simulink model "prelim_plant"  (R2017b)
settings: Solver=VariableStepAuto  StartTime=0.0  StopTime=100  RelTol=1e-3  EnableMultiTasking=on
undefined symbols (not defined in the file or in its folder): A_nom, B_nom, C, D
libraries: cstblocks x6
settings Model: Creator=yyakupog  LastModifiedBy=USER
settings OptimizationCC: LifeSpan=inf
settings DebuggingCC: SFUnexpectedBacktrackingDiag=warning  SFNoUnconditionalDefaultTransitionDiag=warning  SFExecutionAtInitializationDiag=none
settings CodeAppCC: StateflowObjectComments=on
settings GRTTargetCC: TargetLangStandard=C89/C90 (ANSI)  GeneratePreprocessorConditionals=Disable all
settings ConfigComp: CovMetricSettings=dw  CovHtmlReporting=on  CovSaveCumulativeToWorkspaceVar=on  CovSaveSingleToWorkspaceVar=on  CovExternalEMLEnable=off

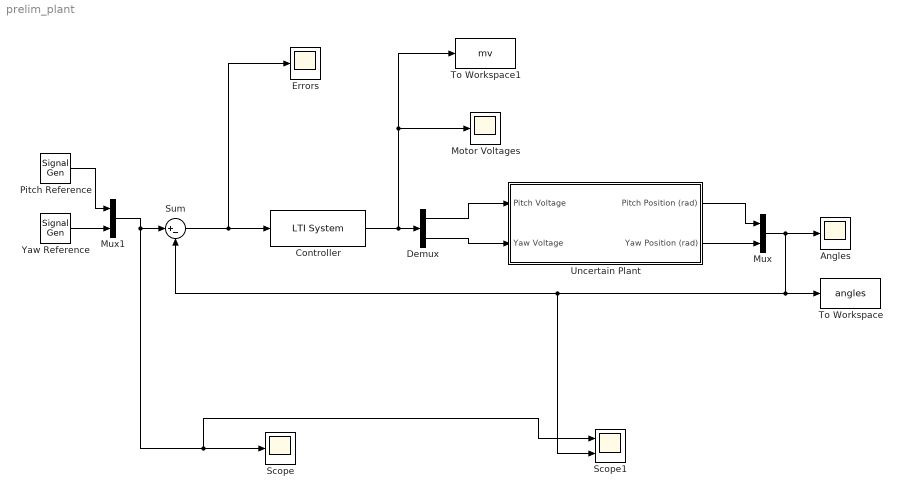
== system prelim_plant ==
  Angles : Scope
  Controller : cstblocks/LTI System  sys=K  IC=[]
  Demux : Demux  Outputs=2
  Errors : Scope
  Motor Voltages : Scope
  Mux : Mux  Inputs=2
  Mux1 : Mux  Inputs=2
  "Pitch Reference " : SignalGenerator  WaveForm=square  Amplitude=pi/6  Frequency=0.4  Units=rad/sec
  Scope : Scope
  Scope1 : Scope  NumInputPorts=2
  Sum : Sum  Inputs=|+-
  To Workspace : ToWorkspace  VariableName=angles  SaveFormat=Timeseries  SampleTime=-1
  To Workspace1 : ToWorkspace  VariableName=mv  SaveFormat=Timeseries  SampleTime=-1
  Uncertain Plant : Subsystem
  Yaw Reference : SignalGenerator  WaveForm=square  Amplitude=pi/4  Frequency=0.5  Units=rad/sec
  wires:
  Controller/1 -> To Workspace1/1, Motor Voltages/1, Demux/1
  Demux/1 -> Uncertain Plant/1(Pitch Voltage)
  Demux/2 -> Uncertain Plant/2(Yaw Voltage)
  Sum/1 -> Errors/1, Controller/1
  Uncertain Plant/1(Pitch Position (rad)) -> Mux/1
  Uncertain Plant/2(Yaw Position (rad)) -> Mux/2
  "Pitch Reference "/1 -> Mux1/1
  Yaw Reference/1 -> Mux1/2
  Mux1/1 -> Scope1/1, Scope/1, Sum/1
  Mux/1 -> To Workspace/1, Scope1/2, Sum/2, Angles/1

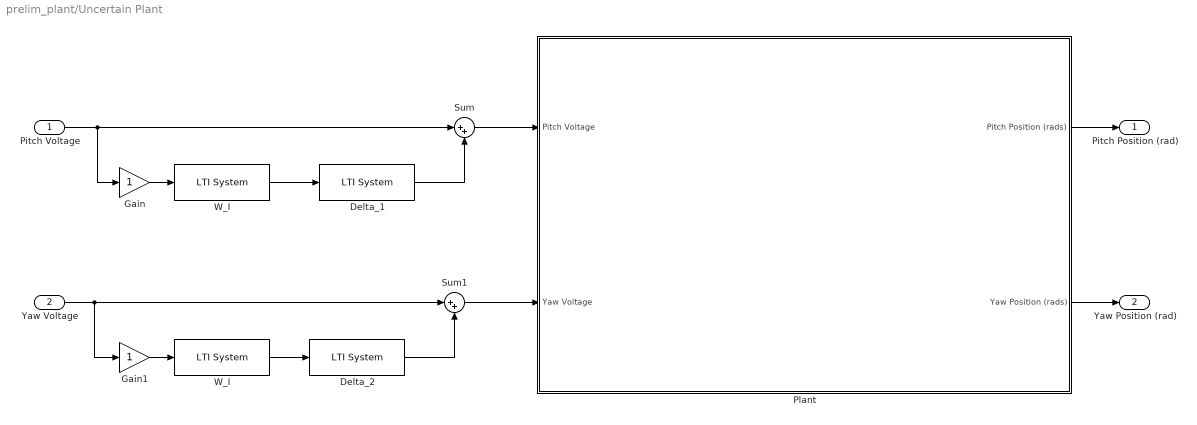
== system prelim_plant/Uncertain Plant ==
  Pitch Voltage : Inport
  Yaw Voltage : Inport  Port=2
  Delta_1 : cstblocks/LTI System  sys=Delta_1  IC=[]
  Delta_2 : cstblocks/LTI System  sys=Delta_2  IC=[]
  Gain : Gain
  Gain1 : Gain
  Plant : Subsystem
  Sum : Sum  Inputs=|++
  Sum1 : Sum  Inputs=|++
  W_I : cstblocks/LTI System  sys=W_I_Pitch  IC=[]
  "W_I " : cstblocks/LTI System  sys=W_I_Yaw  IC=[]
  Pitch Position (rad) : Outport
  Yaw Position (rad) : Outport  Port=2
  wires:
  W_I/1 -> Delta_1/1
  Pitch Voltage/1 -> Sum/1, Gain/1
  Delta_1/1 -> Sum/2
  Yaw Voltage/1 -> Sum1/1, Gain1/1
  Delta_2/1 -> Sum1/2
  "W_I "/1 -> Delta_2/1
  Plant/1(Pitch Position (rads)) -> Pitch Position (rad)/1
  Plant/2(Yaw Position (rads)) -> Yaw Position (rad)/1
  Gain/1 -> W_I/1
  Gain1/1 -> "W_I "/1
  Sum/1 -> Plant/1(Pitch Voltage)
  Sum1/1 -> Plant/2(Yaw Voltage)

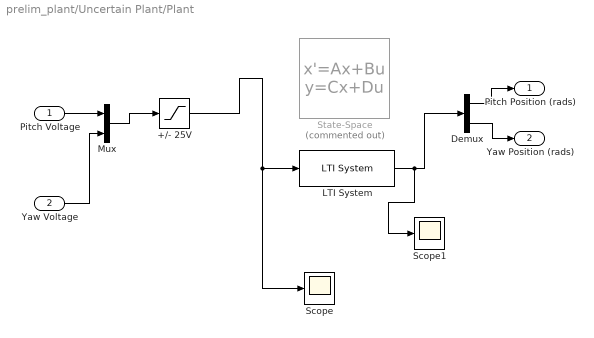
== system prelim_plant/Uncertain Plant/Plant ==
  Pitch Voltage : Inport
  Yaw Voltage : Inport  Port=2
  +/- 25V : Saturate  UpperLimit=25  LowerLimit=-25
  Demux : Demux  Outputs=2
  LTI System : cstblocks/LTI System  sys=G_nom  IC=[]
  Mux : Mux  Inputs=2
  Scope : Scope
  Scope1 : Scope
  State-Space : StateSpace  Commented=on  A=A_nom  B=B_nom  C=C  D=D  InitialCondition=0
  Pitch Position (rads) : Outport
  Yaw Position (rads) : Outport  Port=2
  wires:
  +/- 25V/1 -> Scope/1, LTI System/1
  Pitch Voltage/1 -> Mux/1
  Yaw Voltage/1 -> Mux/2
  Mux/1 -> +/- 25V/1
  Demux/1 -> Pitch Position (rads)/1
  Demux/2 -> Yaw Position (rads)/1
  LTI System/1 -> Scope1/1, Demux/1
